simulink model "qus5"  (R2016a)
settings: Solver=VariableStepAuto  StartTime=0.0  StopTime=50  RelTol=1e-3
undefined symbols (not defined in the file): A, A_5, B, B_5, Br_5, Bw_5, C, C_5, K5, L, y_sp
settings Model: Creator=X1  LastModifiedBy=X1

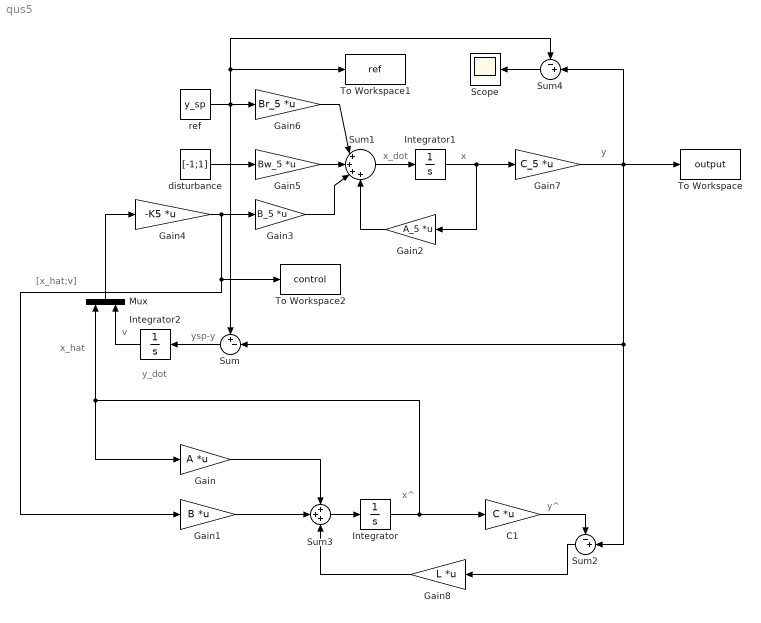
== system qus5 ==
  note: v
  note: [x_hat;v]
  note: y_dot
  note: x_hat
  note: ysp-y
  note: y
  note: x_dot
  note: x
  note: y^
  note: x^
  C1 : Gain  Gain=C  Multiplication=Matrix(K*u)
  Gain : Gain  Gain=A  Multiplication=Matrix(K*u)
  Gain1 : Gain  Gain=B  Multiplication=Matrix(K*u)
  Gain2 : Gain  Gain=A_5  Multiplication=Matrix(K*u)
  Gain3 : Gain  Gain=B_5  Multiplication=Matrix(K*u)
  Gain4 : Gain  Gain=-K5  Multiplication=Matrix(K*u)
  Gain5 : Gain  Gain=Bw_5  Multiplication=Matrix(K*u)
  Gain6 : Gain  Gain=Br_5  Multiplication=Matrix(K*u)
  Gain7 : Gain  Gain=C_5  Multiplication=Matrix(K*u)
  Gain8 : Gain  Gain=L  Multiplication=Matrix(K*u)
  Integrator : Integrator  InitialCondition=[0 0 0 0 0 0]
  Integrator1 : Integrator  InitialCondition=[0 0 0 0 0 0 0 0 0]
  Integrator2 : Integrator  InitialCondition=[0 0 0]
  Mux : Mux  Inputs=2
  Scope : Scope
  Sum : Sum  Inputs=+-|
  Sum1 : Sum  Inputs=|++++
  Sum2 : Sum  Inputs=-+|
  Sum3 : Sum  Inputs=+++
  Sum4 : Sum  Inputs=-+|
  To Workspace : ToWorkspace  VariableName=output  SaveFormat=Timeseries  SampleTime=-1
  To Workspace1 : ToWorkspace  VariableName=ref  SaveFormat=Timeseries  SampleTime=-1
  To Workspace2 : ToWorkspace  VariableName=control  SaveFormat=Timeseries  SampleTime=-1
  disturbance : Constant  Value=[-1;1]
  ref : Constant  Value=y_sp
  wires:
  Integrator1/1 -> Gain2/1, Gain7/1
  Gain2/1 -> Sum1/4
  Gain3/1 -> Sum1/3
  Gain5/1 -> Sum1/2
  disturbance/1 -> Gain5/1
  ref/1 -> Gain6/1, Sum/1, Sum4/1, To Workspace1/1
  Gain6/1 -> Sum1/1
  Sum1/1 -> Integrator1/1
  Mux/1 -> Gain4/1
  Sum/1 -> Integrator2/1
  Integrator2/1 -> Mux/2
  Integrator/1 -> Mux/1, Gain/1, C1/1
  Sum3/1 -> Integrator/1
  Gain4/1 -> To Workspace2/1, Gain1/1, Gain3/1
  C1/1 -> Sum2/1
  Sum2/1 -> Gain8/1
  Gain7/1 -> Sum2/2, Sum/2, Sum4/2, To Workspace/1
  Sum4/1 -> Scope/1
  Gain/1 -> Sum3/1
  Gain1/1 -> Sum3/2
  Gain8/1 -> Sum3/3
